simulink model "systolicArrayWithoutAccumulator"  (R2022b)
settings: Solver=VariableStepAuto  StartTime=0.0  StopTime=10  RelTol=1e-3
libraries: hdlBasic x88, xbsIndex_r4 x1
settings Model: Creator=caval  LastModifiedBy=Heather
settings DebuggingCC: UnconnectedInputMsg=warning  UnconnectedOutputMsg=warning  UnconnectedLineMsg=warning
settings ModelReferenceCC: EnableRefExpFcnMdlSchedulingChecks=on
settings RTWCC: DLArmComputeVersion=19.05

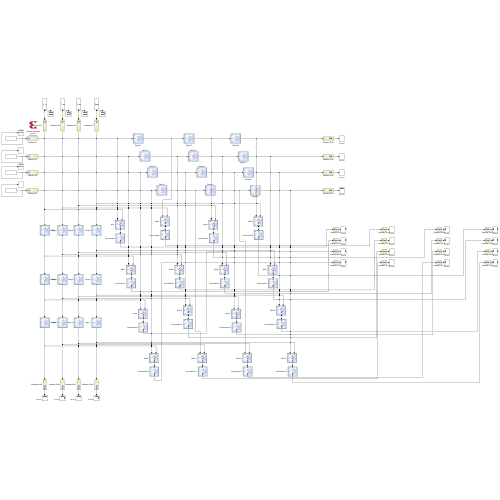
[thumbnail: Simulink's stored preview of the top-level diagram]
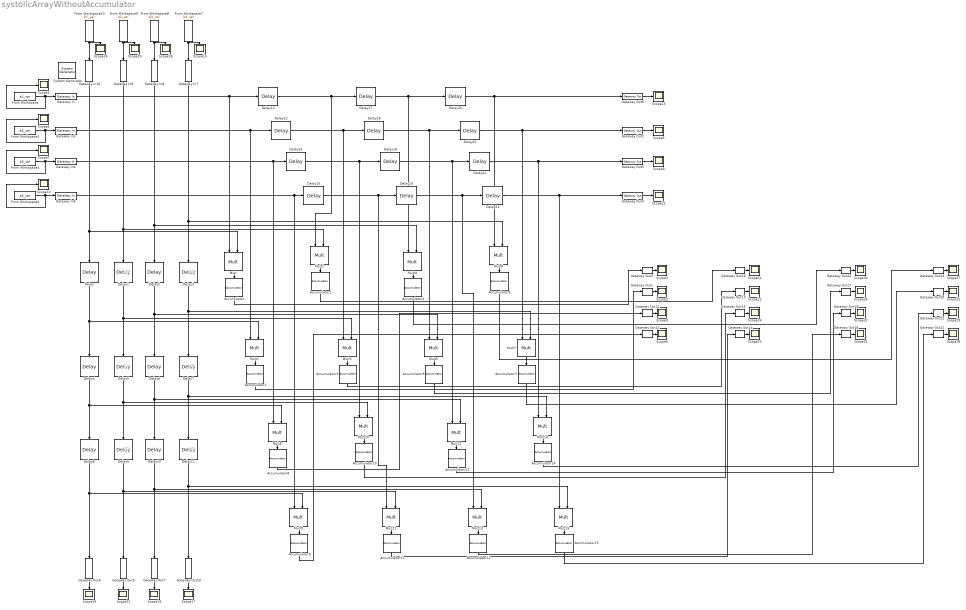
== system systolicArrayWithoutAccumulator ==
  note: 1/2
  note: 1/2
  note: 1/2
  note: 1/2
  note: 1/2
  note: 1/2
  " System Generator" : xbsIndex_r4/ System Generator  Tag=genX  xilinxfamily=zynq  part=xc7z020  speed=-1  package=clg484  synthesis_tool=Vivado  clock_wrapper=Clock Enables  directory=./netlist2  proj_type=Vivado  Synth_file=Vivado Synthesis Defaults  Impl_file=Vivado Implementation Defaults  testbench=off  simulink_period=1  sysclk_period=10  dcm_input_clock_period=10  incr_netlist=off  trim_vbits=Everywhere in SubSystem  dbl_ovrd=According to Block Masks  core_generation=According to Block Masks  run_coregen=off  deprecated_control=off  eval_field=0  block_type=sysgen
  Accumulator{,1..15} (16 alike) : hdlBasic/Accumulator  operation=Add  n_bits=8  overflow=Wrap  scale=1  rst=off  hasbypass=off  en=off  latency=1  msb_inp=100  msb=100  lsb=-100  use_behavioral_HDL=on  implementation=Fabric  XmcBlockStatus=1  maskContainerNames=group3  block_type=accum  block_config=sysgen:Accum_config
  Delay{,1..23} (24 alike) : hdlBasic/Delay  rst=off  en=off  latency=1  reg_retiming=off  XmcBlockStatus=1  maskContainerNames=group1  block_type=delay  block_config=sysgen:Delay_config
  From Workspace : FromWorkspace  VariableName=a1_var
  From Workspace10 : FromWorkspace  VariableName=b1_var
  From Workspace3 : FromWorkspace  VariableName=a2_var
  From Workspace4 : FromWorkspace  VariableName=a3_var
  From Workspace6 : FromWorkspace  VariableName=a4_var
  From Workspace7 : FromWorkspace  VariableName=b4_var
  From Workspace8 : FromWorkspace  VariableName=b3_var
  From Workspace9 : FromWorkspace  VariableName=b2_var
  Gateway In{,3..4,6..10} (8 alike) : hdlBasic/Gateway In  gui_display_data_type=Fixed-point  arith_type=Signed (2's comp)  n_bits=32  bin_pt=0  preci_type=Single  exp_width=8  frac_width=24  rows=1  columns=1  quantization="Round  (unbiased: +/- Inf)"  overflow=Saturate  period=1  UseAsADC=off  ADCChannel='1'  interface=None  automatic_assignment=on  address_offset=hex2dec('00')  intf_name=''  intf_description=''  default_value=0  timing_constraint=None  locs_specified=off  LOCs={}  io_standard={}  inherit_from_input=off  hdl_port=on  XmcBlockStatus=1  maskContainerNames=group4  block_type=gatewayin  block_config=sysgen:gateway_in_config  block_width_w=590  block_height_w=620  block_width=640  block_height=850
  Gateway Out{1..24} (24 alike) : hdlBasic/Gateway Out  inherit_from_input=off  hdl_port=on  rows=1  columns=1  UseAsDAC=off  DACChannel='1'  interface=None  automatic_assignment=on  address_offset=hex2dec('00')  intf_name=''  intf_description=''  timing_constraint=None  locs_specified=off  LOCs={}  io_standard={}  XmcBlockStatus=1  maskContainerNames=group4  block_type=gatewayout  block_config=sysgen:gateway_out_config  block_width_w=590  block_height_w=620  block_width=620  block_height=750
  Mult{,1..15} (16 alike) : hdlBasic/Mult  precision=Full  arith_type="Signed  (2's comp)"  n_bits=16  bin_pt=14  quantization=Truncate  overflow=Wrap  en=off  latency=3  use_behavioral_HDL=off  opt=Speed  use_embedded=on  optimum_pipeline=off  pipeline=on  use_rpm=on  placement_style=Triangular  XmcBlockStatus=1  maskContainerNames=group1  block_type=mult  block_config=sysgen:Mult_config
  Scope{1..32} (32 alike) : Scope
      Scope11 settings: Description=C14  AttributesFormatString=texttest
      Scope12 settings: Description=C14  AttributesFormatString=texttest
      Scope15 settings: Description=C14  AttributesFormatString=texttest
      Scope16 settings: Description=C14  AttributesFormatString=texttest
      Scope17 settings: Description=C14  AttributesFormatString=texttest
      Scope19 settings: Description=C14  AttributesFormatString=texttest
      Scope2 settings: Description=C14  AttributesFormatString=texttest
      Scope21 settings: Description=C14  AttributesFormatString=texttest
      Scope22 settings: Description=C14  AttributesFormatString=texttest
      Scope23 settings: Description=C14  AttributesFormatString=texttest
      Scope24 settings: Description=C14  AttributesFormatString=texttest
      Scope25 settings: Description=C14  AttributesFormatString=texttest
      Scope26 settings: Description=C14  AttributesFormatString=texttest
      Scope27 settings: Description=C14  AttributesFormatString=texttest
      Scope28 settings: Description=C14  AttributesFormatString=texttest
      Scope29 settings: Description=C14  AttributesFormatString=texttest
      Scope3 settings: Description=C14  AttributesFormatString=texttest
      Scope30 settings: Description=C14  AttributesFormatString=texttest
      Scope31 settings: Description=C14  AttributesFormatString=texttest
      Scope32 settings: Description=C14  AttributesFormatString=texttest
      Scope5 settings: Description=C14  AttributesFormatString=texttest
      Scope6 settings: Description=C14  AttributesFormatString=texttest
      Scope8 settings: Description=C14  AttributesFormatString=texttest
      Scope9 settings: Description=C14  AttributesFormatString=texttest
  wires:
  From Workspace/1 -> Scope1/1, Gateway In/1
  Gateway Out6/1 -> Scope15/1
  Mult/1 -> Accumulator/1
  Gateway In/1 -> Delay13/1, Mult/1
  Gateway Out2/1 -> Scope5/1
  From Workspace3/1 -> Scope4/1, Gateway In3/1
  Gateway In3/1 -> Delay12/1, Mult1/1
  From Workspace6/1 -> Scope10/1, Gateway In6/1
  Gateway Out5/1 -> Scope8/1
  Gateway Out4/1 -> Scope11/1
  From Workspace4/1 -> Scope7/1, Gateway In4/1
  Gateway In6/1 -> Delay15/1, Mult9/1
  Gateway In4/1 -> Delay14/1, Mult8/1
  From Workspace8/1 -> Scope18/1, Gateway In8/1
  Gateway Out7/1 -> Scope19/1
  Gateway In9/1 -> Delay1/1, Mult2/2
  Gateway In10/1 -> Delay/1, Mult/2
  Gateway Out8/1 -> Scope16/1
  From Workspace10/1 -> Scope14/1, Gateway In10/1
  Gateway Out10/1 -> Scope17/1
  From Workspace9/1 -> Scope20/1, Gateway In9/1
  Gateway Out9/1 -> Scope21/1
  From Workspace7/1 -> Scope13/1, Gateway In7/1
  Gateway In8/1 -> Delay2/1, Mult4/2
  Gateway In7/1 -> Delay3/1, Mult6/2
  Mult1/1 -> Accumulator1/1
  Delay/1 -> Delay4/1, Mult1/2
  Delay4/1 -> Delay8/1, Mult8/2
  Mult2/1 -> Accumulator2/1
  Delay13/1 -> Delay17/1, Mult2/1
  Mult3/1 -> Accumulator3/1
  Delay12/1 -> Delay16/1, Mult3/1
  Delay1/1 -> Delay5/1, Mult3/2
  Mult7/1 -> Accumulator7/1
  Mult4/1 -> Accumulator4/1
  Mult5/1 -> Accumulator5/1
  Mult6/1 -> Accumulator6/1
  Delay2/1 -> Delay6/1, Mult5/2
  Delay3/1 -> Delay7/1, Mult7/2
  Delay5/1 -> Delay9/1, Mult10/2
  Delay6/1 -> Delay10/1, Mult12/2
  Delay7/1 -> Delay11/1, Mult14/2
  Delay20/1 -> Mult6/1, Gateway Out6/1
  Delay16/1 -> Delay21/1, Mult5/1
  Delay21/1 -> Mult7/1, Gateway Out2/1
  Mult11/1 -> Accumulator11/1
  Mult8/1 -> Accumulator8/1
  Mult15/1 -> Accumulator15/1
  Mult12/1 -> Accumulator12/1
  Mult9/1 -> Accumulator9/1
  Mult10/1 -> Accumulator10/1
  Mult14/1 -> Accumulator14/1
  Mult13/1 -> Accumulator13/1
  Delay8/1 -> Mult9/2, Gateway Out8/1
  Delay11/1 -> Mult15/2, Gateway Out10/1
  Delay9/1 -> Mult11/2, Gateway Out9/1
  Delay10/1 -> Mult13/2, Gateway Out7/1
  Delay18/1 -> Delay22/1, Mult12/1
  Delay22/1 -> Gateway Out5/1, Mult14/1
  Delay19/1 -> Delay23/1, Mult13/1
  Delay23/1 -> Gateway Out4/1, Mult15/1
  Delay14/1 -> Delay18/1, Mult10/1
  Delay15/1 -> Mult11/1, Delay19/1
  Gateway Out3/1 -> Scope3/1
  Delay17/1 -> Delay20/1, Mult4/1
  Accumulator/1 -> Gateway Out3/1
  Gateway Out1/1 -> Scope2/1
  Accumulator1/1 -> Gateway Out1/1
  Gateway Out11/1 -> Scope6/1
  Accumulator9/1 -> Gateway Out11/1
  Gateway Out12/1 -> Scope9/1
  Accumulator8/1 -> Gateway Out12/1
  Accumulator10/1 -> Gateway Out15/1
  Accumulator11/1 -> Gateway Out14/1
  Gateway Out13/1 -> Scope12/1
  Accumulator3/1 -> Gateway Out13/1
  Gateway Out14/1 -> Scope23/1
  Gateway Out16/1 -> Scope22/1
  Accumulator2/1 -> Gateway Out16/1
  Gateway Out15/1 -> Scope24/1
  Gateway Out22/1 -> Scope29/1
  Accumulator6/1 -> Gateway Out23/1
  Gateway Out21/1 -> Scope28/1
  Gateway Out20/1 -> Scope25/1
  Accumulator14/1 -> Gateway Out22/1
  Accumulator12/1 -> Gateway Out19/1
  Accumulator13/1 -> Gateway Out18/1
  Gateway Out23/1 -> Scope27/1
  Accumulator7/1 -> Gateway Out20/1
  Accumulator15/1 -> Gateway Out21/1
  Gateway Out17/1 -> Scope26/1
  Accumulator5/1 -> Gateway Out17/1
  Gateway Out18/1 -> Scope31/1
  Gateway Out24/1 -> Scope30/1
  Accumulator4/1 -> Gateway Out24/1
  Gateway Out19/1 -> Scope32/1
